simulink model "Blocked_Rotor_Test"  (R2025a)
settings: Solver=ode23tb  StartTime=0.0  StopTime=5  MaxStep=1e-4  RelTol=1e-3
libraries: spsCurrentMeasurementLib x3, spsACVoltageSourceLib x3, spsVoltageMeasurementLib x3, spsRMSLib x2, spsAsynchronousMachineSIUnitsLib x1, spsPower3phInstantaneousLib x1, sps_lib x1
settings Model: Creator=Jawad  LastModifiedBy=Jawad

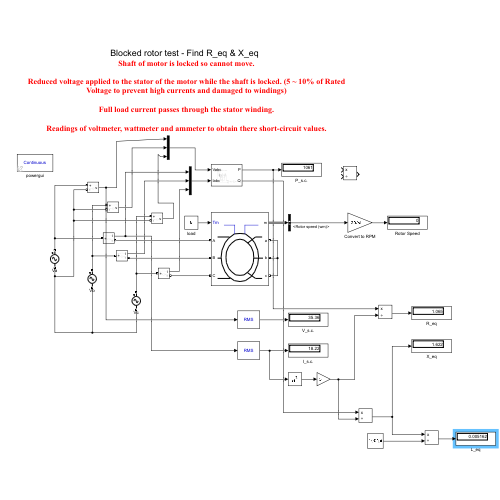
[thumbnail: Simulink's stored preview of the top-level diagram]
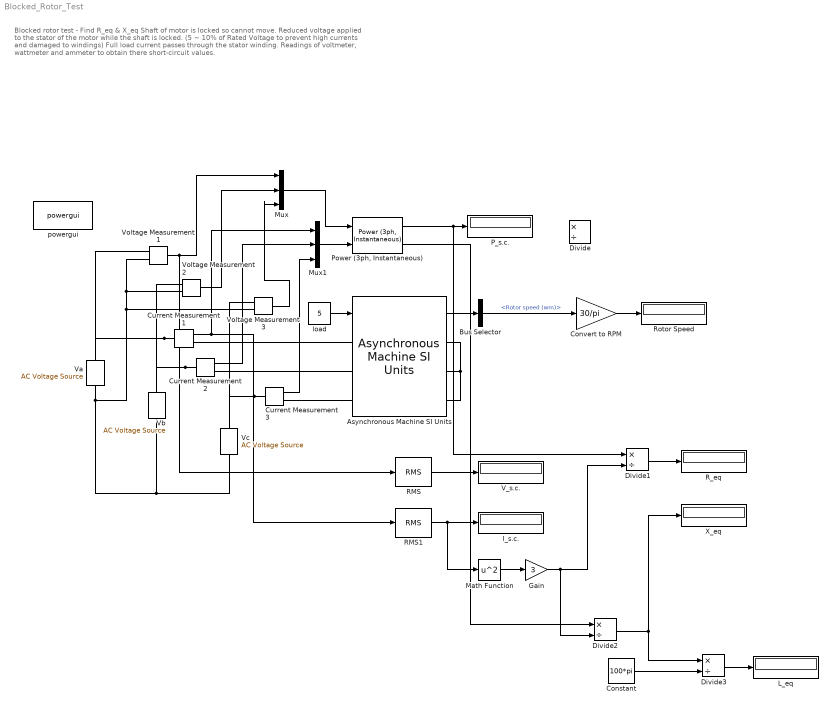
== system Blocked_Rotor_Test ==
  note: Blocked rotor test - Find R_eq & X_eq
      | Shaft of motor is locked so cannot move.
      |
      | Reduced voltage applied to the stator of the motor while the shaft is locked. (5 ~ 10% of Rated Voltage to prevent high currents and damaged to windings)
      |
      | Full load current passes through the stator winding.
      |
      | Readings of voltmeter, wattmeter and ammeter to obtain there short-circuit values.
  Asynchronous Machine SI Units : spsAsynchronousMachineSIUnitsLib/Asynchronous Machine SI Units  RotorType=Wound  PresetModel=No  MechanicalLoad=Torque Tm  ShowDetailedParameters=on  ReferenceFrame=Rotor  Units=SI  MeasurementBus=off  NominalParameters=[1.845e+04 460 50]  VoltageRatio=1  Stator=[0.5968 0.0003495]  Rotor=[0.6258 0.005473]  Cage1=[0.4155 0.002066]  Cage2=[0.4168 0.0003495]  Lm=0.0354  Mechanical=[inf 0.005879 2]  PolePairs=2  InitialConditions=[1 0 0 0 0 0 0 0]  SimulateSaturation=off  Saturation=[14.03593122, 27.81365428, 53.79336849, 72.68890987, 97.98006896, 148.6815601, 215.7428561, 302.9841135, 428.7778367 ; 230, 322, 414, 460, 506, 552, 598, 644, 690]  LoadFlowParameters=1492000  TsPowergui=0  TsBlock=-1  IterativeModel=Trapezoidal non iterative  IterativeDiscreteModel=Trapezoidal non iterative  Pmec=1.492e+006
  Bus Selector : BusSelector  OutputSignals=Mechanical.Rotor speed (wm)
  Constant : Constant  Value=100*pi
  Convert to RPM : Gain  Gain=30/pi
  Current Measurement1 : spsCurrentMeasurementLib/Current Measurement  PhasorSimulation=off  OutputType=Complex  PSBequivalent=0
  Current Measurement2 : spsCurrentMeasurementLib/Current Measurement  PhasorSimulation=off  OutputType=Complex  PSBequivalent=0
  Current Measurement3 : spsCurrentMeasurementLib/Current Measurement  PhasorSimulation=off  OutputType=Complex  PSBequivalent=0
  Divide{,1..3} (4 alike) : Product  Inputs=*/
  Gain : Gain  Gain=3
  I_s.c. : Display
  L_eq : Display
  Math Function : Math  Operator=square
  Mux : Mux  Inputs=3
  Mux1 : Mux  Inputs=3
  P_s.c. : Display
  "Power (3ph, Instantaneous)" : spsPower3phInstantaneousLib/Power (3ph, Instantaneous)
  RMS : spsRMSLib/RMS  TrueRMS=on  Freq=50  RMSInit=0  Ts=0
  RMS1 : spsRMSLib/RMS  TrueRMS=on  Freq=50  RMSInit=0  Ts=0
  R_eq : Display
  Rotor Speed : Display
  V_s.c. : Display
  Va : spsACVoltageSourceLib/AC Voltage Source  Amplitude=50  Phase=0  Frequency=50  SampleTime=0  Measurements=None  BusType=swing  Pref=10e3  Qref=0  Qmin=-inf  Qmax=+inf
  Vb : spsACVoltageSourceLib/AC Voltage Source  Amplitude=50  Phase=-120  Frequency=50  SampleTime=0  Measurements=None  BusType=swing  Pref=10e3  Qref=0  Qmin=-inf  Qmax=+inf
  Vc : spsACVoltageSourceLib/AC Voltage Source  Amplitude=50  Phase=120  Frequency=50  SampleTime=0  Measurements=None  BusType=swing  Pref=10e3  Qref=0  Qmin=-inf  Qmax=+inf
  Voltage Measurement1 : spsVoltageMeasurementLib/Voltage Measurement  PhasorSimulation=off  OutputType=Complex  PSBequivalent=0
  Voltage Measurement2 : spsVoltageMeasurementLib/Voltage Measurement  PhasorSimulation=off  OutputType=Complex  PSBequivalent=0
  Voltage Measurement3 : spsVoltageMeasurementLib/Voltage Measurement  PhasorSimulation=off  OutputType=Complex  PSBequivalent=0
  X_eq : Display
  load : Constant  Value=5
  powergui : sps_lib/powergui  Priority=1  SimulationMode=Continuous  SampleTime=50e-6  frequency=60  Iterations=50  frequencyindice=50  Pbase=100e6  ErrMax=1e-4  UnitsV=kV  UnitsW=MW  buscounter=0  FunctionMessages=off  echomessages=off  EnableUseOfTLC=off  CurrentSourceSwitches=off  DisableSnubberDevices=off  DisableRonSwitches=off  DisableVfSwitches=off  DisplayEquations=off  AutomaticDiscreteSolvers=off  SolverType=Tustin/Backward Euler (TBE)  Interpol=off  ExternalGateDelay=off  methode=off  Ts=100  x0status=blocks  SPID=on  SwTol=0  HookPort=off  NonlinearTolerance=1e-4  nMaxIteration=100  ContinueOnMaxIteration=off  RestoreLinks=warning  ResistiveCurrentMeasurement=off  Frange=[0:2:500]  Ylog=off  Xlog=on  ShowGrid=off  save=off  variable=ZData  structure=0  ZoomFFT=off  StartTime=0.0  cycles=1  DisplayStyle=1  fundamental=60  FreqAxis=off  MaxFrequency=1000  frequencyindicesteady=1  RmsSteady=1  display=off
  wires:
  Bus Selector/1 -> Convert to RPM/1  "<Rotor speed (wm)>"
  Current Measurement2/1 -> Mux1/2
  Convert to RPM/1 -> Rotor Speed/1
  RMS1/1 -> Math Function/1, I_s.c./1
  Mux1/1 -> "Power (3ph, Instantaneous)"/2
  Current Measurement3/1 -> Mux1/3
  Voltage Measurement2/1 -> Mux/2
  RMS/1 -> V_s.c./1
  Current Measurement1/1 -> RMS1/1, Mux1/1
  Mux/1 -> "Power (3ph, Instantaneous)"/1
  Asynchronous Machine SI Units/1 -> Bus Selector/1
  "Power (3ph, Instantaneous)"/1 -> Divide1/1, P_s.c./1
  Voltage Measurement1/1 -> RMS/1, Mux/1
  load/1 -> Asynchronous Machine SI Units/1
  Voltage Measurement3/1 -> Mux/3
  Math Function/1 -> Gain/1
  Divide1/1 -> R_eq/1
  Gain/1 -> Divide2/2, Divide1/2
  Divide2/1 -> Divide3/1, X_eq/1
  "Power (3ph, Instantaneous)"/2 -> Divide2/1
  Constant/1 -> Divide3/2
  Divide3/1 -> L_eq/1
  connections:
  Voltage Measurement1/LConn2 -- Voltage Measurement3/LConn2 -- Vc/LConn1 -- Vb/LConn1 -- Va/LConn1 -- Voltage Measurement2/LConn2
  Current Measurement1/LConn1 -- Voltage Measurement1/LConn1 -- Va/RConn1
  Current Measurement3/LConn1 -- Vc/RConn1 -- Voltage Measurement3/LConn1
  Current Measurement2/LConn1 -- Vb/RConn1 -- Voltage Measurement2/LConn1
  Asynchronous Machine SI Units/RConn2 -- Asynchronous Machine SI Units/RConn1 -- Asynchronous Machine SI Units/RConn3
  Current Measurement2/RConn1 -- Asynchronous Machine SI Units/LConn2
  Current Measurement1/RConn1 -- Asynchronous Machine SI Units/LConn1
  Current Measurement3/RConn1 -- Asynchronous Machine SI Units/LConn3
